simulink model "FINAL_SUBMISSION_REORGANIZED_A1 (1)"  (R2022b)
settings: Solver=FixedStepAuto  StartTime=0.0  StopTime=10.0  FixedStep=1e-3  RelTol=1e-3  EnableMultiTasking=on
undefined symbols (not defined in the file): D0, D1, D10, D11, D12, D13, D2, D3, D4, D5, D6, D7, D8, D9, PTA0, PTA1, PTA2, PTB23, PTB9, PTC16, PTC17, PTC2, PTC3, PTC4, PTD0, PTD1, PTD2, PTD3
libraries: frdmk64flib x16
settings Model: ExtModeTrigDuration=5  Creator=sonja  LastModifiedBy=Quinn Gauder
settings SolverCC: AlgebraicLoopSolver=TrustRegion
settings OptimizationCC: EnhancedBackFolding=on  PassReuseOutputArgsAs=Individual arguments  ZeroExternalMemoryAtStartup=off  ZeroInternalMemoryAtStartup=off  MaxStackSize=64  OptimizeBlockOrder=speed  DifferentSizesBufferReuse=on  OptimizationCustomize=off  EfficientTunableParamExpr=on
settings DebuggingCC: ParameterTunabilityLossMsg=error  UnconnectedInputMsg=warning  UnconnectedOutputMsg=warning  UnconnectedLineMsg=warning  SFMachineParentedDataDiag=warning
settings HardwareCC: ProdBitPerPointer=32  ProdBitPerSizeT=32  ProdBitPerPtrDiffT=32  ProdLargestAtomicInteger=Long  ProdLargestAtomicFloat=Double  ProdWordSize=32  ProdHWDeviceType=ARM Compatible->ARM Cortex
settings ModelReferenceCC: EnableRefExpFcnMdlSchedulingChecks=on
settings SFSimCC: MATLABDynamicMemAlloc=off
settings RTWCC: Description=Embedded Coder  SystemTargetFile=ert.tlc  HardwareBoard=NXP FRDM-K64F  TLCOptions="-aInlineSetEventsForThisBaseRateFcn=TLC_FALSE -aSuppressMultiTaskScheduler=TLC_FALSE  -aRateBasedStepFcn=0"  TemplateMakefile=ert_default_tmf  Toolchain=GNU Tools for ARM Embedded Processors  DLArmComputeVersion=19.05
settings CodeAppCC: ForceParamTrailComments=on  IgnoreCustomStorageClasses=off  OperatorAnnotations=on  SimulinkDataObjDesc=on  SFDataObjDesc=on  InsertBlockDesc=on
settings ERTTargetCC: ExtModeTransport=4  ExtModeMexFile=sendToCommService

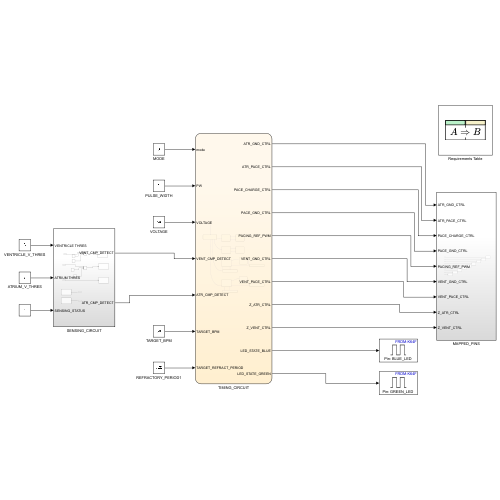
[thumbnail: Simulink's stored preview of the top-level diagram]
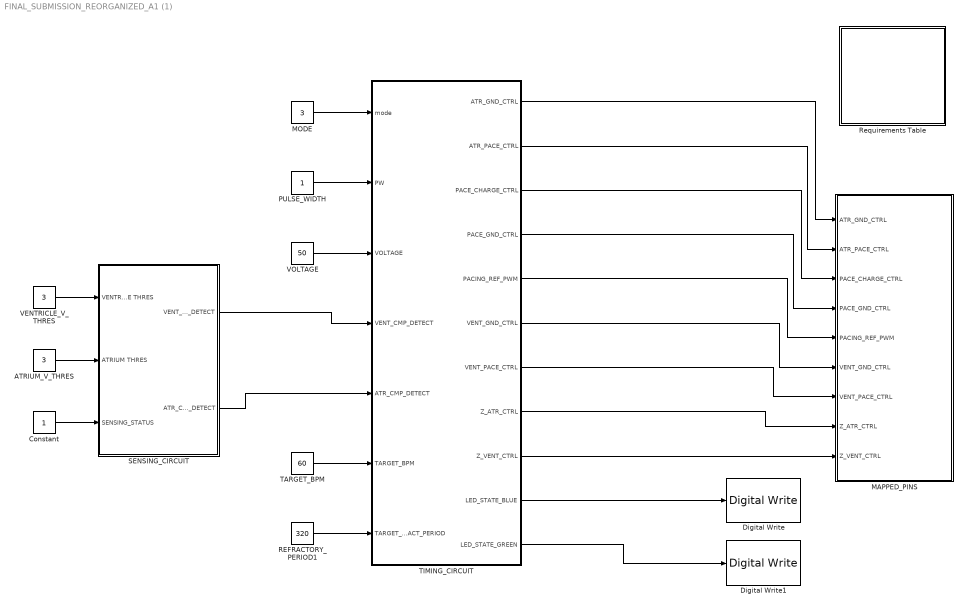
== system FINAL_SUBMISSION_REORGANIZED_A1 (1) ==
  ATRIUM_V_THRES : Constant  Value=3  OutDataTypeStr=int16
  Constant : Constant  OutDataTypeStr=int16
  Digital Write : frdmk64flib/Digital Write  Whichpin=BLUE_LED
  Digital Write1 : frdmk64flib/Digital Write  Whichpin=GREEN_LED
  MAPPED_PINS : Subsystem
  MODE : Constant  Value=3  OutDataTypeStr=int16
  PULSE_WIDTH : Constant  OutDataTypeStr=int16
  REFRACTORY_PERIOD1 : Constant  Value=320  OutDataTypeStr=int16
  Requirements Table : Requirements Table  TreatAsAtomicUnit=on
  SENSING_CIRCUIT : Subsystem
  TARGET_BPM : Constant  Value=60  OutDataTypeStr=int16
  TIMING_CIRCUIT : Stateflow chart  TreatAsAtomicUnit=on
  VENTRICLE_V_THRES : Constant  Value=3  OutDataTypeStr=int16
  VOLTAGE : Constant  Value=50  OutDataTypeStr=int16
  wires:
  PULSE_WIDTH/1 -> TIMING_CIRCUIT/2(PW)
  VOLTAGE/1 -> TIMING_CIRCUIT/3(VOLTAGE)
  TIMING_CIRCUIT/1(ATR_GND_CTRL) -> MAPPED_PINS/1(ATR_GND_CTRL)
  TIMING_CIRCUIT/2(ATR_PACE_CTRL) -> MAPPED_PINS/2(ATR_PACE_CTRL)
  TIMING_CIRCUIT/3(PACE_CHARGE_CTRL) -> MAPPED_PINS/3(PACE_CHARGE_CTRL)
  TIMING_CIRCUIT/4(PACE_GND_CTRL) -> MAPPED_PINS/4(PACE_GND_CTRL)
  TIMING_CIRCUIT/5(PACING_REF_PWM) -> MAPPED_PINS/5(PACING_REF_PWM)
  TIMING_CIRCUIT/6(VENT_GND_CTRL) -> MAPPED_PINS/6(VENT_GND_CTRL)
  TIMING_CIRCUIT/7(VENT_PACE_CTRL) -> MAPPED_PINS/7(VENT_PACE_CTRL)
  TIMING_CIRCUIT/8(Z_ATR_CTRL) -> MAPPED_PINS/8(Z_ATR_CTRL)
  TIMING_CIRCUIT/9(Z_VENT_CTRL) -> MAPPED_PINS/9(Z_VENT_CTRL)
  TIMING_CIRCUIT/10(LED_STATE_BLUE) -> Digital Write/1
  TIMING_CIRCUIT/11(LED_STATE_GREEN) -> Digital Write1/1
  VENTRICLE_V_THRES/1 -> SENSING_CIRCUIT/1(VENTRICLE THRES)
  ATRIUM_V_THRES/1 -> SENSING_CIRCUIT/2(ATRIUM THRES)
  SENSING_CIRCUIT/1(VENT_CMP_DETECT) -> TIMING_CIRCUIT/4(VENT_CMP_DETECT)
  SENSING_CIRCUIT/2(ATR_CMP_DETECT) -> TIMING_CIRCUIT/5(ATR_CMP_DETECT)
  MODE/1 -> TIMING_CIRCUIT/1(mode)
  TARGET_BPM/1 -> TIMING_CIRCUIT/6(TARGET_BPM)
  Constant/1 -> SENSING_CIRCUIT/3(SENSING_STATUS)
  REFRACTORY_PERIOD1/1 -> TIMING_CIRCUIT/7(TARGET_REFRACT_PERIOD)

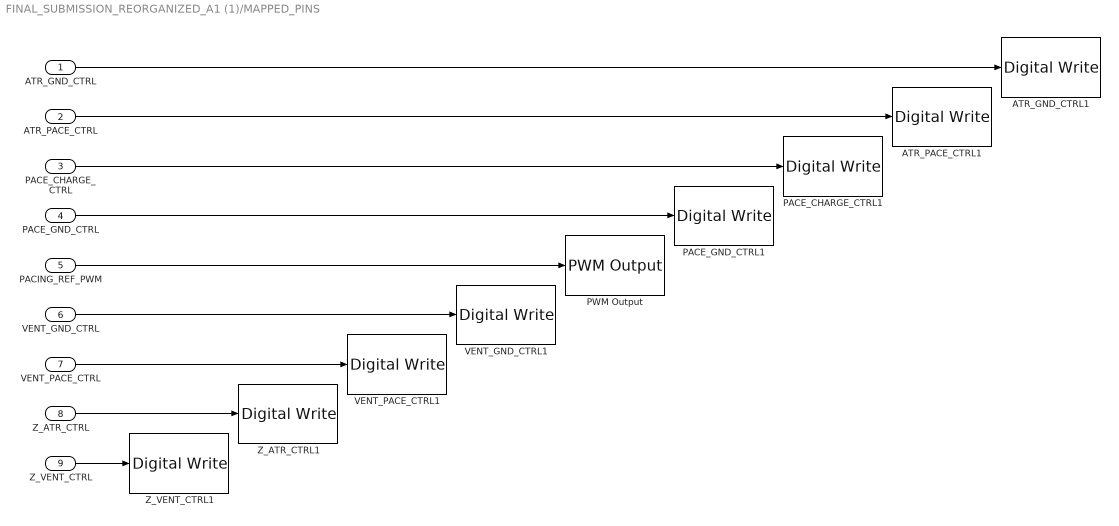
== system FINAL_SUBMISSION_REORGANIZED_A1 (1)/MAPPED_PINS ==
  ATR_GND_CTRL : Inport
  ATR_PACE_CTRL : Inport  Port=2
  PACE_CHARGE_CTRL : Inport  Port=3
  PACE_GND_CTRL : Inport  Port=4
  PACING_REF_PWM : Inport  Port=5
  VENT_GND_CTRL : Inport  Port=6
  VENT_PACE_CTRL : Inport  Port=7
  Z_ATR_CTRL : Inport  Port=8
  Z_VENT_CTRL : Inport  Port=9
  ATR_GND_CTRL1 : frdmk64flib/Digital Write  Whichpin=PTD2 (D11)
  ATR_PACE_CTRL1 : frdmk64flib/Digital Write  Whichpin=PTA0 (D8)
  PACE_CHARGE_CTRL1 : frdmk64flib/Digital Write  Whichpin=PTB9 (D2)
  PACE_GND_CTRL1 : frdmk64flib/Digital Write  Whichpin=PTD0 (D10)
  PWM Output : frdmk64flib/PWM Output  Whichpin=PTA2 (D5)  InitialFrequency=2000  InitialDutyCycle=0
  VENT_GND_CTRL1 : frdmk64flib/Digital Write  Whichpin=PTD3 (D12)
  VENT_PACE_CTRL1 : frdmk64flib/Digital Write  Whichpin=PTC4 (D9)
  Z_ATR_CTRL1 : frdmk64flib/Digital Write  Whichpin=PTB23 (D4)
  Z_VENT_CTRL1 : frdmk64flib/Digital Write  Whichpin=PTC3 (D7)
  wires:
  ATR_GND_CTRL/1 -> ATR_GND_CTRL1/1
  ATR_PACE_CTRL/1 -> ATR_PACE_CTRL1/1
  PACE_CHARGE_CTRL/1 -> PACE_CHARGE_CTRL1/1
  PACE_GND_CTRL/1 -> PACE_GND_CTRL1/1
  PACING_REF_PWM/1 -> PWM Output/1
  VENT_GND_CTRL/1 -> VENT_GND_CTRL1/1
  VENT_PACE_CTRL/1 -> VENT_PACE_CTRL1/1
  Z_ATR_CTRL/1 -> Z_ATR_CTRL1/1
  Z_VENT_CTRL/1 -> Z_VENT_CTRL1/1

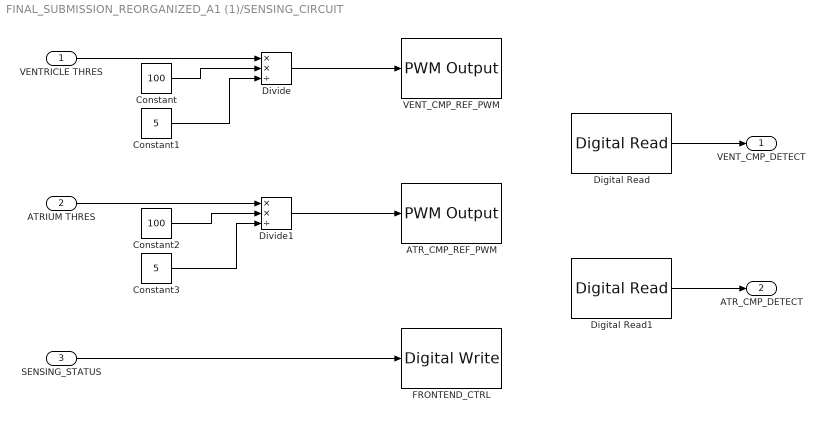
== system FINAL_SUBMISSION_REORGANIZED_A1 (1)/SENSING_CIRCUIT ==
  VENTRICLE THRES : Inport  OutDataTypeStr=int16
  ATRIUM THRES : Inport  Port=2  OutDataTypeStr=int16
  SENSING_STATUS : Inport  Port=3  OutDataTypeStr=int16
  ATR_CMP_REF_PWM : frdmk64flib/PWM Output  Whichpin=PTC2 (D6)  InitialFrequency=2000  InitialDutyCycle=0
  Constant : Constant  Value=100  OutDataTypeStr=int16
  Constant1 : Constant  Value=5  OutDataTypeStr=single
  Constant2 : Constant  Value=100  OutDataTypeStr=int16
  Constant3 : Constant  Value=5  OutDataTypeStr=single
  Digital Read : frdmk64flib/Digital Read  Whichpin=PTC17 (D1)  SampleTime=-1
  Digital Read1 : frdmk64flib/Digital Read  Whichpin=PTC16 (D0)  SampleTime=-1
  Divide : Product  Inputs=**/  OutDataTypeStr=single
  Divide1 : Product  Inputs=**/  OutDataTypeStr=single
  FRONTEND_CTRL : frdmk64flib/Digital Write  Whichpin=PTD1 (D13)
  VENT_CMP_REF_PWM : frdmk64flib/PWM Output  Whichpin=PTA1 (D3)  InitialFrequency=2000  InitialDutyCycle=0
  VENT_CMP_DETECT : Outport  OutDataTypeStr=boolean
  ATR_CMP_DETECT : Outport  Port=2  OutDataTypeStr=boolean
  wires:
  ATRIUM THRES/1 -> Divide1/1
  Constant/1 -> Divide/2
  VENTRICLE THRES/1 -> Divide/1
  Constant1/1 -> Divide/3
  Constant2/1 -> Divide1/2
  Constant3/1 -> Divide1/3
  Divide/1 -> VENT_CMP_REF_PWM/1
  Divide1/1 -> ATR_CMP_REF_PWM/1
  Digital Read1/1 -> ATR_CMP_DETECT/1
  Digital Read/1 -> VENT_CMP_DETECT/1
  SENSING_STATUS/1 -> FRONTEND_CTRL/1

== stateflow chart FINAL_SUBMISSION_REORGANIZED_A1 (1)/Requirements Table ==
  (default) -> (junction 1073741860)
  (junction 1073741860) -> (junction 1073741861) : {
      | % SF_REQ_REV_07
      | }
  (junction 1073741861) -> (junction 1073741863) : {
      | % HEADER_ASSIGNMENTS
      |
      | }
  (junction 1073741863) -> (junction 1073741865) : {
      | % START_A_4
      | }
  (junction 1073741865) -> (junction 1073741867) : {
      | }
  (junction 1073741867) -> (junction 1073741869)
  (junction 1073741869) -> (junction 1073741871) : {
      | }
  (junction 1073741871) -> (junction 1073741873) : {
      | % END_A_4
      | }
  (junction 1073741873) -> (junction 1073741898) : {
      | % START_R_1
      | }
  (junction 1073741898) -> (junction 1073741900) : {
      | }
  (junction 1073741900) -> (junction 1073741902) : {
      |
      |
      | }
  (junction 1073741902) -> (junction 1073741904) : {
      | }
  (junction 1073741904) -> (junction 1073741906) : {
      | % END_R_1
      | }

== stateflow chart FINAL_SUBMISSION_REORGANIZED_A1 (1)/TIMING_CIRCUIT ==
  state Main
    entry:
    %where variables are set for hardware hiding
    LRI = 1000;
    VENT_REFRACTORY_PERIOD = TARGET_REFRACT_PERIOD;
    ATR_REFRACTORY_PERIOD = TARGET_REFRACT_PERIOD;
  state CHARGING_C22_VENTRICLE
    entry:
    LED_STATE_GREEN = true;
    LED_STATE_BLUE = false;
    PACE_CHARGE_CTRL = true;
    PACE_GND_CTRL = true;
    VENT_PACE_CTRL = false;
    Z_ATR_CTRL = false;
    Z_VENT_CTRL = false;
    ATR_PACE_CTRL = false;
    VENT_GND_CTRL = true;
    PACING_REF_PWM = VOLTAGE;
  state DISCHARGE_C22_VENTRICLE
    entry:
    LED_STATE_GREEN = false;
    LED_STATE_BLUE = true;
    PACE_GND_CTRL = true;
    VENT_PACE_CTRL = true;
    Z_ATR_CTRL = false;
    Z_VENT_CTRL = false;
    ATR_PACE_CTRL = false;
    ATR_GND_CTRL = false;
    VENT_GND_CTRL = false;
  state CHARGING_C22_ATRIUM
    entry:
    LED_STATE_GREEN = true;
    LED_STATE_BLUE = false;
    PACE_CHARGE_CTRL = true;
    PACE_GND_CTRL = true;
    VENT_PACE_CTRL = false;
    Z_ATR_CTRL = false;
    Z_VENT_CTRL = false;
    ATR_PACE_CTRL = false;
    VENT_GND_CTRL = false;
    ATR_GND_CTRL = true;
    PACING_REF_PWM = VOLTAGE;
  state DISCHARGE_C22_ATRIUM
    entry:
    LED_STATE_GREEN = false;
    LED_STATE_BLUE = true;
    PACE_GND_CTRL = true;
    VENT_PACE_CTRL = false;
    Z_ATR_CTRL = false;
    Z_VENT_CTRL = false;
    ATR_PACE_CTRL = true;
    ATR_GND_CTRL = false;
    VENT_GND_CTRL = false;
  state DISCHARGING
    entry:
    LED_STATE_GREEN = false;
    LED_STATE_BLUE = true;
    PACE_GND_CTRL = true;
    VENT_PACE_CTRL = true;
    Z_ATR_CTRL = false;
    Z_VENT_CTRL = false;
    ATR_PACE_CTRL = false;
    ATR_GND_CTRL = false;
    VENT_GND_CTRL = false;
  state CHARGING1
    entry:
    LED_STATE_GREEN = true;
    LED_STATE_BLUE = false;
    PACE_CHARGE_CTRL = true;
    PACE_GND_CTRL = true;
    VENT_PACE_CTRL = false;
    Z_ATR_CTRL = false;
    Z_VENT_CTRL = false;
    ATR_PACE_CTRL = false;
    VENT_GND_CTRL = true;
    PACING_REF_PWM = VOLTAGE;
  state SENSING3
    LRI=((60000/TARGET_BPM)-PW);
    VENT_REFRACTORY_PERIOD=TARGET_REFRACT_PERIOD-PW;
  state SENSING
    VENT_REFRACTORY_PERIOD = TARGET_REFRACT_PERIOD;
    LRI=60000/TARGET_BPM;
  state DISCHARGE_C22_ATRIUM1
    entry:
    LED_STATE_GREEN = false;
    LED_STATE_BLUE = true;
    PACE_GND_CTRL = true;
    VENT_PACE_CTRL = false;
    Z_ATR_CTRL = false;
    Z_VENT_CTRL = false;
    ATR_PACE_CTRL = true;
    ATR_GND_CTRL = false;
    VENT_GND_CTRL = false;
  state CHARGING_C22_ATRIUM1
    entry:
    LED_STATE_GREEN = true;
    LED_STATE_BLUE = false;
    PACE_CHARGE_CTRL = true;
    PACE_GND_CTRL = true;
    VENT_PACE_CTRL = false;
    Z_ATR_CTRL = false;
    Z_VENT_CTRL = false;
    ATR_PACE_CTRL = false;
    VENT_GND_CTRL = false;
    ATR_GND_CTRL = true;
    PACING_REF_PWM = VOLTAGE;
  state SENSING2
    LRI=((60000/TARGET_BPM)-PW);
    ATR_REFRACTORY_PERIOD=TARGET_REFRACT_PERIOD-PW;
  state SENSING1
    ATR_REFRACTORY_PERIOD = TARGET_REFRACT_PERIOD;
    LRI=60000/TARGET_BPM;
  (default) -> Main
  CHARGING_C22_VENTRICLE -> DISCHARGE_C22_VENTRICLE : after(LRI - PW,msec)
  Main -> CHARGING_C22_VENTRICLE [order 1] : [mode == 1] %VOO
  DISCHARGE_C22_VENTRICLE -> CHARGING_C22_VENTRICLE : after(PW,msec)
  Main -> SENSING1 [order 4] : after(ATR_REFRACTORY_PERIOD,msec)[mode==4] %AAI
  Main -> SENSING [order 3] : after(VENT_REFRACTORY_PERIOD,msec)[mode == 3] %VVI
  Main -> CHARGING_C22_ATRIUM [order 2] : [mode == 2] %AOO
  CHARGING_C22_ATRIUM -> DISCHARGE_C22_ATRIUM : after(LRI-PW,msec)
  DISCHARGE_C22_ATRIUM -> CHARGING_C22_ATRIUM : after(PW,msec)
  CHARGING1 -> DISCHARGING [order 1] : after(LRI-PW,msec)
  DISCHARGING -> SENSING3 : after(PW,msec)
  SENSING3 -> CHARGING1
  SENSING -> CHARGING1
  CHARGING1 -> SENSING [order 2] : after(VENT_REFRACTORY_PERIOD,msec)[VENT_CMP_DETECT == true]
  CHARGING_C22_ATRIUM1 -> DISCHARGE_C22_ATRIUM1 [order 1] : after(LRI-PW,msec)
  DISCHARGE_C22_ATRIUM1 -> SENSING2 : after(PW,msec)
  SENSING2 -> CHARGING_C22_ATRIUM1
  SENSING1 -> CHARGING_C22_ATRIUM1
  CHARGING_C22_ATRIUM1 -> SENSING1 [order 2] : after(ATR_REFRACTORY_PERIOD,msec)[ATR_CMP_DETECT==true]
  data: mode input int16; ATR_GND_CTRL output boolean; ATR_PACE_CTRL output boolean; PACE_CHARGE_CTRL output boolean; PACE_GND_CTRL output boolean; PACING_REF_PWM output int16; PW input int16; VENT_GND_CTRL output boolean; VENT_PACE_CTRL output boolean; VOLTAGE input int16; Z_ATR_CTRL output boolean; Z_VENT_CTRL output boolean; LED_STATE_BLUE output boolean; LED_STATE_GREEN output boolean; VENT_CMP_DETECT input boolean; ATR_CMP_DETECT input boolean; TARGET_BPM input int16; LRI local int16; VENT_REFRACTORY_PERIOD local; TARGET_REFRACT_PERIOD input int16; ATR_REFRACTORY_PERIOD local
